simulink model "lab_1_qpsk_lpf_z"  (Simulink 7.5)
settings: Solver=ode45  StartTime=0.0  StopTime=0.000045  FixedStep=Td  RelTol=1e-3
values from neighbouring files (symbols this model uses):
  Fc = 2*pi*Rs    (= 2814867.01762)    [lab_1_parameters.m]
  Rb = Nvar*64000    (= 896000)    [lab_1_parameters.m]
  Td = Ts/128    (= 1.74386160714e-08)    [lab_1_parameters.m]
  Ts = 1/Rs    (= 2.23214285714e-06)    [lab_1_parameters.m]
undefined symbols (not defined in the file or in its folder): dfilt, figposition, Fs
libraries: dspsrcs4 x4, dsparch4 x4, dspsnks4 x4, commsink2 x3, commrandsrc2 x2, simulink x2, commdigbbndpm2 x2, commchan3 x1
settings Model: Creator=alex  LastModifiedBy=alex
settings OptimizationCC: InlineInvariantSignals=on  InitFltsAndDblsToZero=on
settings DebuggingCC: SaveWithParameterizedLinksMsg=none  SignalResolutionControl=TryResolveAllWithWarning  MultiTaskDSMMsg=warning  MultiTaskCondExecSysMsg=none  StrictBusMsg=None
settings RTWCC: IncludeERTFirstTime=on
settings GRTTargetCC: TargetFcnLib=ansi_tfl_tmw.mat

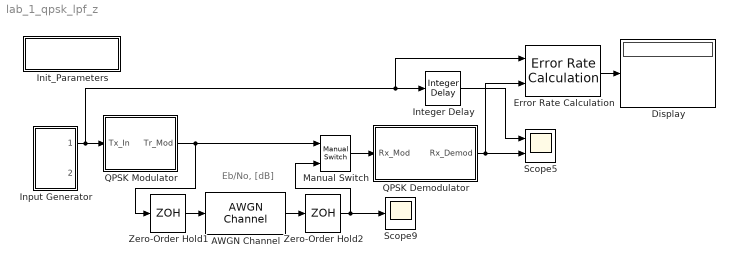
== system lab_1_qpsk_lpf_z ==
  note: Eb/No, [dB]
  AWGN Channel : commchan3/AWGN Channel  SystemSampleTime=-1  seed=56479  noiseMode="Signal to noise ratio  (Eb/No)"  EbNodB=EbNodB  EsNodB=15  SNRdB=10  bitsPerSym=2  Ps=1  Tsym=Ts  variance=1
  Display : Display
  Error Rate Calculation : commsink2/Error Rate Calculation  N=2  st_delay=0  cp_mode=Entire frame  subframe=[]  PMode=Port  WsName=ErrorVec  RsMode2=off  stop=off  numErr=100  maxBits=1e6
  Init_Parameters : Subsystem
      settings: OpenFcn=lab_1_parameters
      mask Display: disp('lab_1_parameters')
  Input Generator : Subsystem
  Integer Delay : simulink/Discrete/Integer Delay  vinit=0.0  samptime=-1  NumDelays=2
  Manual Switch : simulink/Signal Routing/Manual Switch  SystemSampleTime=-1  sw=1  action=0  varsize=off
  QPSK Demodulator : Subsystem
  QPSK Modulator : Subsystem
  Scope5 : Scope  NumInputPorts=2
      settings: TimeRange=5  YMin=-5~-5  YMax=5~5  SaveName=ScopeData5
  Scope9 : Scope
      settings: SaveName=ScopeData9
  Zero-Order Hold1 : ZeroOrderHold  SampleTime=Td
  Zero-Order Hold2 : ZeroOrderHold  SampleTime=Td
  wires:
  Error Rate Calculation/1 -> Display/1
  QPSK Modulator/1(Tr_Mod) -> Manual Switch/1, Zero-Order Hold1/1
  Manual Switch/1 -> QPSK Demodulator/1(Rx_Mod)
  Input Generator/1(Integer) -> QPSK Modulator/1(Tx_In), Integer Delay/1, Error Rate Calculation/1
  QPSK Demodulator/1(Rx_Demod) -> Error Rate Calculation/2, Scope5/2
  AWGN Channel/1 -> Zero-Order Hold2/1
  Zero-Order Hold1/1 -> AWGN Channel/1
  Zero-Order Hold2/1 -> Manual Switch/2, Scope9/1
  Integer Delay/1 -> Scope5/1

== system lab_1_qpsk_lpf_z/Init_Parameters ==

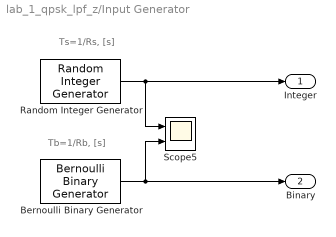
== system lab_1_qpsk_lpf_z/Input Generator ==
  note: Ts=1/Rs, [s]
  note: Tb=1/Rb, [s]
  Bernoulli Binary Generator : commrandsrc2/Bernoulli Binary Generator  DialogController=commDDGCreate  DialogControllerArgs=DataTag0  SystemSampleTime=-1  P=0.5  seed=12345  Ts=1/Rb  frameBased=off  sampPerFrame=1  orient=off  outDataType=double
  Random Integer Generator : commrandsrc2/Random Integer Generator  SystemSampleTime=-1  mul=4  seed=21435  Ts=Ts  frameBased=off  sampPerFrame=1  orient=off  outDataType=double
  Scope5 : Scope  NumInputPorts=2
      settings: TimeRange=5  YMin=-5~-5  YMax=5~5  SaveName=ScopeData11
  Integer : Outport  OutDataType=sfix(16)  OutScaling=2^0
  Binary : Outport  Port=2  OutDataType=sfix(16)  OutScaling=2^0
  wires:
  Random Integer Generator/1 -> Integer/1, Scope5/1
  Bernoulli Binary Generator/1 -> Scope5/2, Binary/1

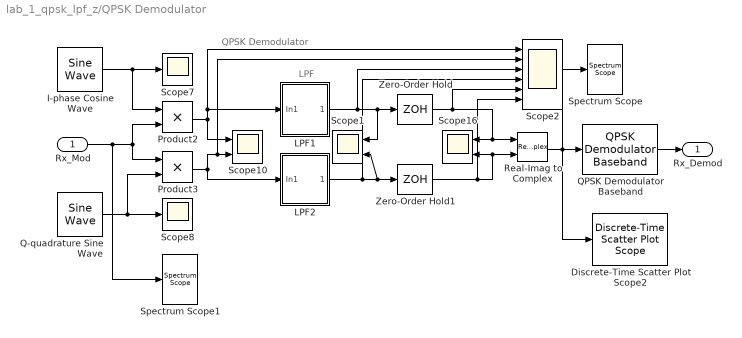
== system lab_1_qpsk_lpf_z/QPSK Demodulator ==
  note: LPF
  note: QPSK Demodulator
  Rx_Mod : Inport  OutDataType=sfix(16)  OutScaling=2^0
  Discrete-Time Scatter Plot Scope2 : commsink2/Discrete-Time Scatter Plot Scope  Tag=ScatterPlot  SystemSampleTime=-1  sampPerSymb=1  offsetEye=0  numTraces=40  numNewFrames=10  LineMarkers=.  LineColors=b  fading=on  render=on  AxisGrid=on  xMin=-1.5  xMax=1.5  yMin=-1.5  yMax=1.5  inphaseLabel=In-phase Amplitude  quadratureLabel=Quadrature Amplitude  openScopeAtSimStart=on  FrameNumber=off  FigPos=[360 138 560 560]  figTitle=Scatter Plot  numLinesMax=8  block_type_=scatter
  I-phase Cosine Wave : dspsrcs4/Sine Wave  Amplitude=sqrt(2)  Frequency=Fc  Phase=pi/2  SampleMode=Discrete  OutComplex=Real  CompMethod=Trigonometric fcn  TableSize=Speed  SampleTime=Td  SamplesPerFrame=1  dataType=double  wordLen=16  udDataType=sfix(16)  fracBitsMode=Best precision  numFracBits=15  ResetState=Restart at time zero
  LPF1 : Subsystem
  LPF2 : Subsystem
  Product2 : Product  OutDataType=sfix(16)  OutScaling=2^0  RndMeth=Zero
  Product3 : Product  OutDataType=sfix(16)  OutScaling=2^0  RndMeth=Zero
  Q-quadrature Sine Wave : dspsrcs4/Sine Wave  Amplitude=sqrt(2)  Frequency=Fc  Phase=pi  SampleMode=Discrete  OutComplex=Real  CompMethod=Trigonometric fcn  TableSize=Speed  SampleTime=Td  SamplesPerFrame=1  dataType=double  wordLen=16  udDataType=sfix(16)  fracBitsMode=Best precision  numFracBits=15  ResetState=Restart at time zero
  QPSK Demodulator Baseband : commdigbbndpm2/QPSK Demodulator Baseband  SystemSampleTime=-1  OutType=Integer  Dec=Binary  Ph=pi/4  numSamp=1
  Real-Imag to Complex : RealImagToComplex
  Scope1 : Scope  NumInputPorts=2
      settings: YMin=-5~-5  YMax=5~5  SaveName=ScopeData4
  Scope10 : Scope  NumInputPorts=2
      settings: YMin=-5~-5  YMax=5~5  SaveName=ScopeData10
  Scope16 : Scope  NumInputPorts=2
      settings: YMin=-5~-5  YMax=5~5
  Scope2 : Scope  NumInputPorts=6
      settings: YMin=-5~-5~-5~-5~-5~-5  YMax=5~5~5~5~5~5  SaveName=ScopeData12
  Scope7 : Scope
      settings: SaveName=ScopeData7
  Scope8 : Scope
      settings: SaveName=ScopeData8
  Spectrum Scope : dspsnks4/Spectrum Scope  DialogController=dspdialog.SpectrumScope  DialogControllerArgs=DataTag5  SystemSampleTime=-1  ScopeProperties=on  Domain=Frequency  HorizSpan=1  UseBuffer=on  BufferSize=256  Overlap=0  inpFftLenInherit=off  FFTlength=128  numAvg=20  DisplayProperties=off  AxisGrid=on  Memory=off  FrameNumber=off  AxisLegend=off  AxisZoom=off  OpenScopeAtSimStart=off  OpenScopeImmediately=off  FigPos="figposition([49    12    39    27])"  AxisProperties=off  XUnits=Hertz  XRange=[-Fs/2...Fs/2]  XDisplay=0  InheritXIncr=on  XIncr=1.0  XLabel=Samples  XLimit=Auto  YUnits=dB  XMax=1  XMin=0  YLabel=Magnitude-squared, dB  LineProperties=off  LineColors=[1 0 0]  wintypeSpecScope=Hann  RsSpecScope=50  betaSpecScope=5  winsampSpecScope=Periodic  XAxisParamsVer=6.8
      settings: YMin=-10  YMax=10
  Spectrum Scope1 : dspsnks4/Spectrum Scope  DialogController=dspdialog.SpectrumScope  DialogControllerArgs=DataTag6  SystemSampleTime=-1  ScopeProperties=on  Domain=Frequency  HorizSpan=1  UseBuffer=on  BufferSize=256  Overlap=0  inpFftLenInherit=off  FFTlength=128  numAvg=20  DisplayProperties=off  AxisGrid=on  Memory=off  FrameNumber=off  AxisLegend=off  AxisZoom=off  OpenScopeAtSimStart=on  OpenScopeImmediately=off  FigPos="figposition([49    12    39    27])"  AxisProperties=off  XUnits=Hertz  XRange=[-Fs/2...Fs/2]  XDisplay=0  InheritXIncr=on  XIncr=1.0  XLabel=Samples  XLimit=Auto  YUnits=dBW/Hertz  XMax=1  XMin=0  YLabel=Magnitude-squared, dB  LineProperties=off  LineColors=[1 0 0]  wintypeSpecScope=Hann  RsSpecScope=50  betaSpecScope=5  winsampSpecScope=Periodic  XAxisParamsVer=6.8
      settings: YMin=-87.5849  YMax=-67.5849
  Zero-Order Hold : ZeroOrderHold  SampleTime=Ts
  Zero-Order Hold1 : ZeroOrderHold  SampleTime=Ts
  Rx_Demod : Outport  OutDataType=sfix(16)  OutScaling=2^0
  wires:
  I-phase Cosine Wave/1 -> Scope7/1, Product2/1
  Q-quadrature Sine Wave/1 -> Scope8/1, Product3/2
  Real-Imag to Complex/1 -> QPSK Demodulator Baseband/1, Spectrum Scope/1, Discrete-Time Scatter Plot Scope2/1
  Rx_Mod/1 -> Product2/2, Product3/1, Spectrum Scope1/1
  QPSK Demodulator Baseband/1 -> Rx_Demod/1
  LPF1/1(Out1) -> Zero-Order Hold/1, Scope1/1, Scope2/3
  Product3/1 -> LPF2/1(In1), Scope10/2, Scope2/2
  Product2/1 -> Scope10/1, LPF1/1(In1), Scope2/1
  LPF2/1(Out1) -> Zero-Order Hold1/1, Scope1/2, Scope2/4
  Zero-Order Hold/1 -> Real-Imag to Complex/1, Scope16/1, Scope2/5
  Zero-Order Hold1/1 -> Real-Imag to Complex/2, Scope16/2, Scope2/6

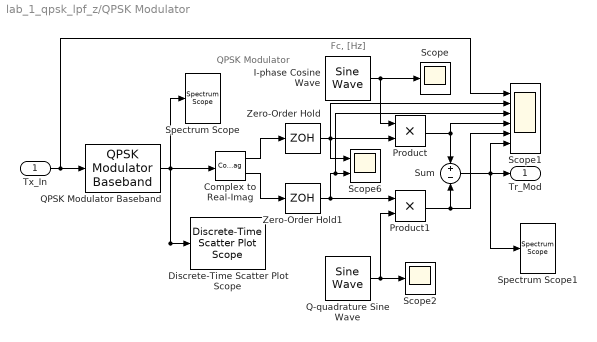
== system lab_1_qpsk_lpf_z/QPSK Modulator ==
  note: QPSK Modulator
  note: Fc, [Hz]
  Tx_In : Inport  OutDataType=sfix(16)  OutScaling=2^0
  Complex to Real-Imag : ComplexToRealImag
  Discrete-Time Scatter Plot Scope : commsink2/Discrete-Time Scatter Plot Scope  Tag=ScatterPlot  SystemSampleTime=-1  sampPerSymb=1  offsetEye=0  numTraces=40  numNewFrames=10  LineMarkers=.  LineColors=b  fading=on  render=on  AxisGrid=on  xMin=-1.5  xMax=1.5  yMin=-1.5  yMax=1.5  inphaseLabel=In-phase Amplitude  quadratureLabel=Quadrature Amplitude  openScopeAtSimStart=on  FrameNumber=off  FigPos=[360 138 560 560]  figTitle=Scatter Plot  numLinesMax=8  block_type_=scatter
  I-phase Cosine Wave : dspsrcs4/Sine Wave  Amplitude=sqrt(2)  Frequency=Fc  Phase=pi/2  SampleMode=Discrete  OutComplex=Real  CompMethod=Trigonometric fcn  TableSize=Speed  SampleTime=Td  SamplesPerFrame=1  dataType=double  wordLen=16  udDataType=sfix(16)  fracBitsMode=Best precision  numFracBits=15  ResetState=Restart at time zero
  Product : Product  OutDataType=sfix(16)  OutScaling=2^0  RndMeth=Zero
  Product1 : Product  OutDataType=sfix(16)  OutScaling=2^0  RndMeth=Zero
  Q-quadrature Sine Wave : dspsrcs4/Sine Wave  Amplitude=1  Frequency=Fc  Phase=0  SampleMode=Discrete  OutComplex=Real  CompMethod=Trigonometric fcn  TableSize=Speed  SampleTime=Td  SamplesPerFrame=1  dataType=double  wordLen=16  udDataType=sfix(16)  fracBitsMode=Best precision  numFracBits=15  ResetState=Restart at time zero
  QPSK Modulator Baseband : commdigbbndpm2/QPSK Modulator Baseband  SystemSampleTime=-1  InType=Integer  Enc=Binary  Ph=pi/4  numSamp=1
  Scope : Scope
      settings: SaveName=ScopeData2
  Scope1 : Scope  NumInputPorts=6
      settings: TimeRange=5  YMin=-5~-5~-5~-5~-5~-5  YMax=5~5~5~5~5~5
  Scope2 : Scope
      settings: SaveName=ScopeData3
  Scope6 : Scope  NumInputPorts=2
      settings: YMin=-5~-5  YMax=5~5  SaveName=ScopeData6
  Spectrum Scope : dspsnks4/Spectrum Scope  DialogController=dspdialog.SpectrumScope  DialogControllerArgs=DataTag7  SystemSampleTime=-1  ScopeProperties=on  Domain=Frequency  HorizSpan=1  UseBuffer=on  BufferSize=256  Overlap=0  inpFftLenInherit=off  FFTlength=128  numAvg=20  DisplayProperties=off  AxisGrid=on  Memory=off  FrameNumber=off  AxisLegend=off  AxisZoom=off  OpenScopeAtSimStart=off  OpenScopeImmediately=off  FigPos="figposition([49    12    39    27])"  AxisProperties=off  XUnits=Hertz  XRange=[-Fs/2...Fs/2]  XDisplay=0  InheritXIncr=on  XIncr=1.0  XLabel=Samples  XLimit=Auto  YUnits=dB  XMax=1  XMin=0  YLabel=Magnitude-squared, dB  LineProperties=off  LineColors=[1 0 0]  wintypeSpecScope=Hann  RsSpecScope=50  betaSpecScope=5  winsampSpecScope=Periodic  XAxisParamsVer=6.8
      settings: YMin=-10  YMax=10
  Spectrum Scope1 : dspsnks4/Spectrum Scope  DialogController=dspdialog.SpectrumScope  DialogControllerArgs=DataTag8  SystemSampleTime=-1  ScopeProperties=on  Domain=Frequency  HorizSpan=1  UseBuffer=on  BufferSize=256  Overlap=0  inpFftLenInherit=off  FFTlength=128  numAvg=20  DisplayProperties=off  AxisGrid=on  Memory=off  FrameNumber=off  AxisLegend=off  AxisZoom=off  OpenScopeAtSimStart=on  OpenScopeImmediately=off  FigPos="figposition([49    12    39    27])"  AxisProperties=off  XUnits=Hertz  XRange=[-Fs/2...Fs/2]  XDisplay=0  InheritXIncr=on  XIncr=1.0  XLabel=Samples  XLimit=Auto  YUnits=dBW/Hertz  XMax=1  XMin=0  YLabel=Magnitude-squared, dB  LineProperties=off  LineColors=[1 0 0]  wintypeSpecScope=Hann  RsSpecScope=50  betaSpecScope=5  winsampSpecScope=Periodic  XAxisParamsVer=6.8
      settings: YMin=-87.5849  YMax=-67.5849
  Sum : Sum  Inputs=+-  OutDataType=sfix(16)  OutScaling=2^0
  Zero-Order Hold : ZeroOrderHold  SampleTime=Ts
  Zero-Order Hold1 : ZeroOrderHold  SampleTime=Ts
  Tr_Mod : Outport  OutDataType=sfix(16)  OutScaling=2^0
  wires:
  Product1/1 -> Sum/2, Scope1/5
  QPSK Modulator Baseband/1 -> Complex to Real-Imag/1, Discrete-Time Scatter Plot Scope/1, Spectrum Scope/1
  Product/1 -> Sum/1, Scope1/4
  Sum/1 -> Tr_Mod/1, Spectrum Scope1/1, Scope1/6
  Tx_In/1 -> QPSK Modulator Baseband/1, Scope1/1
  Complex to Real-Imag/2 -> Zero-Order Hold1/1
  Complex to Real-Imag/1 -> Zero-Order Hold/1
  Zero-Order Hold1/1 -> Product1/1, Scope6/2, Scope1/3
  I-phase Cosine Wave/1 -> Product/1, Scope/1
  Q-quadrature Sine Wave/1 -> Product1/2, Scope2/1
  Zero-Order Hold/1 -> Product/2, Scope6/1, Scope1/2

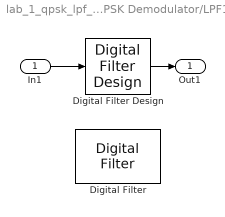
== system lab_1_qpsk_lpf_z/QPSK Demodulator/LPF1 ==
  In1 : Inport  OutDataType=sfix(16)  OutScaling=2^0
  Digital Filter Design : dsparch4/Digital Filter Design  SystemSampleTime=-1  mwdsp_browser_bugfix_var=off
  Digital Filter : dsparch4/Digital Filter  DialogController=dspdialog.DigitalFilter  DialogControllerArgs=DataTag2  TypePopup=FIR (all zeros)  IIRFiltStruct=Direct form II transposed  AllPoleFiltStruct=Direct form  FIRFiltStruct=Direct form  CoeffSource=Specify via dialog  NumCoeffs=[1 2]  DenCoeffs=[1 0.1]  BiQuadCoeffs=[1 0.3 0.4 1 0.1 0.2]  LatticeCoeffs=[0.2 0.4]  denIgnore=on  FiltPerSampPopup=One filter per frame  IC=0  ICnum=0  ICden=0  roundingMode=Floor  overflowMode=off  ScaleValues=1  scaleValueFracLength=14  stageInFracLength=15  stageOutFracLength=15  FilterSource=Specify via dialog  dfiltObjectName=dfilt.dffir([1 2 1])
  Out1 : Outport  OutDataType=sfix(16)  OutScaling=2^0
  wires:
  In1/1 -> Digital Filter Design/1
  Digital Filter Design/1 -> Out1/1

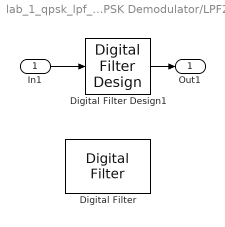
== system lab_1_qpsk_lpf_z/QPSK Demodulator/LPF2 ==
  In1 : Inport  OutDataType=sfix(16)  OutScaling=2^0
  Digital Filter Design1 : dsparch4/Digital Filter Design  SystemSampleTime=-1  mwdsp_browser_bugfix_var=off
  Digital Filter : dsparch4/Digital Filter  DialogController=dspdialog.DigitalFilter  DialogControllerArgs=DataTag4  TypePopup=IIR (poles & zeros)  IIRFiltStruct=Direct form II transposed  AllPoleFiltStruct=Direct form  FIRFiltStruct=Direct form  CoeffSource=Specify via dialog  NumCoeffs=[1 2]  DenCoeffs=[1 0.1]  BiQuadCoeffs=[1 0.3 0.4 1 0.1 0.2]  LatticeCoeffs=[0.2 0.4]  denIgnore=on  FiltPerSampPopup=One filter per frame  IC=0  ICnum=0  ICden=0  roundingMode=Floor  overflowMode=off  ScaleValues=1  scaleValueFracLength=14  stageInFracLength=15  stageOutFracLength=15  FilterSource=Specify via dialog  dfiltObjectName=dfilt.dffir([1 2 1])
  Out1 : Outport  OutDataType=sfix(16)  OutScaling=2^0
  wires:
  In1/1 -> Digital Filter Design1/1
  Digital Filter Design1/1 -> Out1/1
